simulink model "SingleWksWithTimeBasedFailures"  (R2015a)
settings: Solver=ode45  StartTime=0.0  StopTime=100000  RelTol=1e-3
InitFcn:
  | se_randomizeseeds(gcs, 'Mode', 'All')
undefined symbols (not defined in the file): se_randomizeseeds
libraries: simeventslib x8
settings Model: CovSFcnEnable=off  Creator=gthiers3  LastModifiedBy=gthiers3
settings DebuggingCC: SolverPrmCheckMsg=warning

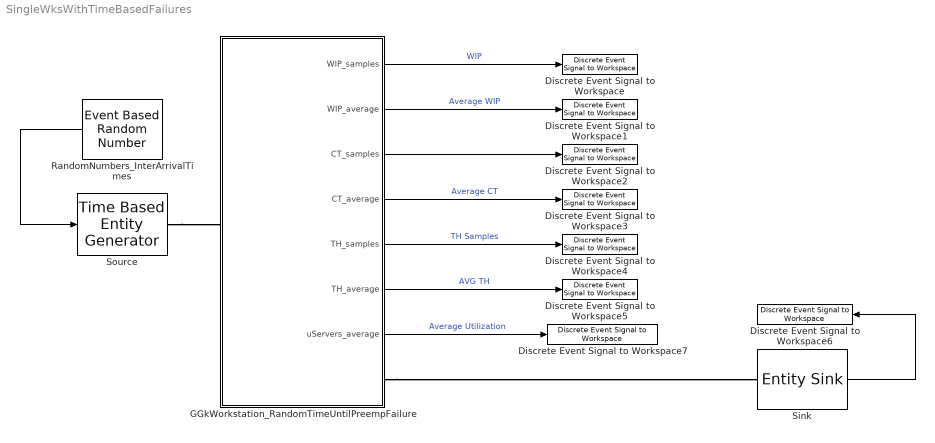
== system SingleWksWithTimeBasedFailures ==
  Discrete Event Signal to Workspace : simeventslib/SimEvents Sinks/Discrete Event Signal to Workspace  VariableName=WIP_samples  SaveFormat=Structure With Time  isMonitorOnly=off  isRecordIC=off
  Discrete Event Signal to Workspace1 : simeventslib/SimEvents Sinks/Discrete Event Signal to Workspace  VariableName=WIP_average  SaveFormat=Structure With Time  isMonitorOnly=off  isRecordIC=off
  Discrete Event Signal to Workspace2 : simeventslib/SimEvents Sinks/Discrete Event Signal to Workspace  VariableName=CT_samples  SaveFormat=Structure With Time  isMonitorOnly=off  isRecordIC=off
  Discrete Event Signal to Workspace3 : simeventslib/SimEvents Sinks/Discrete Event Signal to Workspace  VariableName=CT_average  SaveFormat=Structure With Time  isMonitorOnly=off  isRecordIC=off
  Discrete Event Signal to Workspace4 : simeventslib/SimEvents Sinks/Discrete Event Signal to Workspace  VariableName=TH_samples  SaveFormat=Structure With Time  isMonitorOnly=off  isRecordIC=off
  Discrete Event Signal to Workspace5 : simeventslib/SimEvents Sinks/Discrete Event Signal to Workspace  VariableName=TH_average  SaveFormat=Structure With Time  isMonitorOnly=off  isRecordIC=off
  Discrete Event Signal to Workspace6 : simeventslib/SimEvents Sinks/Discrete Event Signal to Workspace  VariableName=nDepartures  SaveFormat=Structure With Time  isMonitorOnly=off  isRecordIC=off
  Discrete Event Signal to Workspace7 : simeventslib/SimEvents Sinks/Discrete Event Signal to Workspace  VariableName=uServers_average  SaveFormat=Structure With Time  isMonitorOnly=off  isRecordIC=off
  GGkWorkstation_RandomTimeUntilPreempFailure : Subsystem  InitFcn=se_randomizeseeds(gcs, 'Mode', 'All')
      settings: CopyFcn=set_param(gcb, 'LinkStatus', 'none');
  RandomNumbers_InterArrivalTimes : EventBasedRandomNumber  meanExp=25  scaleGam=10  meanNorm=100  stdNorm=eps  Seed=41684
  Sink : EntitySink  StatNumberArrived=on
  Source : TimeBasedEntityGenerator  GenerateEntitiesUpon=Intergeneration time from port t
  wires:
  RandomNumbers_InterArrivalTimes/1 -> Source/1
  GGkWorkstation_RandomTimeUntilPreempFailure/1(WIP_samples) -> Discrete Event Signal to Workspace/1  "WIP"
  GGkWorkstation_RandomTimeUntilPreempFailure/2(WIP_average) -> Discrete Event Signal to Workspace1/1  "Average WIP"
  GGkWorkstation_RandomTimeUntilPreempFailure/3(CT_samples) -> Discrete Event Signal to Workspace2/1
  GGkWorkstation_RandomTimeUntilPreempFailure/4(CT_average) -> Discrete Event Signal to Workspace3/1  "Average CT"
  GGkWorkstation_RandomTimeUntilPreempFailure/7(uServers_average) -> Discrete Event Signal to Workspace7/1  "Average Utilization"
  GGkWorkstation_RandomTimeUntilPreempFailure/6(TH_average) -> Discrete Event Signal to Workspace5/1  "AVG TH"
  GGkWorkstation_RandomTimeUntilPreempFailure/5(TH_samples) -> Discrete Event Signal to Workspace4/1  "TH Samples"
  Sink/1 -> Discrete Event Signal to Workspace6/1
  connections:
  Source/RConn1 -- GGkWorkstation_RandomTimeUntilPreempFailure/LConn1
  GGkWorkstation_RandomTimeUntilPreempFailure/RConn1 -- Sink/LConn1

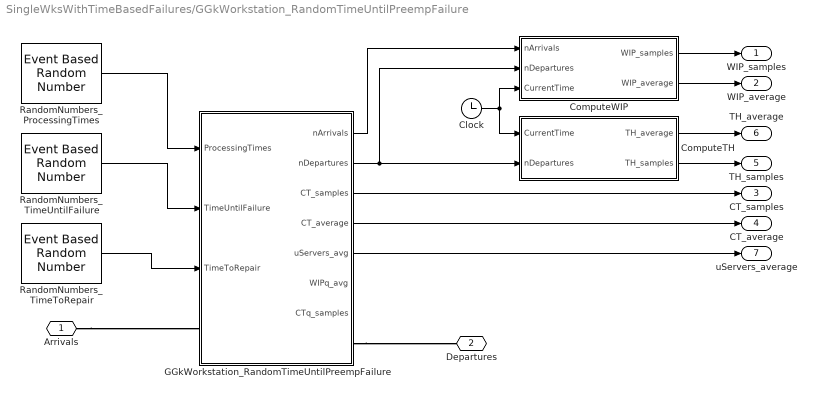
== system SingleWksWithTimeBasedFailures/GGkWorkstation_RandomTimeUntilPreempFailure ==
  Clock : Clock
  ComputeTH : Subsystem
  ComputeWIP : Subsystem
  GGkWorkstation_RandomTimeUntilPreempFailure : Subsystem  mask{NumberOfServers=1}
      mask prompts: NumberOfServers "Number of servers:"
      mask TypeOptions NumberOfServers: N-Server/NumberOfServers
      mask DialogControl DescTextVar Prompt: GG1 Workstation, with random time intervals until preemptive failure and random repair times.  Timing is consistent with Hopp & Spearman’s model, in that the time-until-failure clock stops during repair.
  RandomNumbers_ProcessingTimes : EventBasedRandomNumber  Distribution=Triangular  meanExp=15  minUnif=40  maxUnif=40  pOneBern=40  pSuccessBino=40  numTrialBino=40  minTri=5  maxTri=25  modeTri=15  thresholdGam=40  scaleGam=40  shapeGam=40  meanNorm=95  stdNorm=eps  pSuccessGeo=40  meanPoiss=40  thresholdLogn=40  scaleLogn=40  shapeLogn=40  thresholdLogl=40  scaleLogl=40  minBeta=40  maxBeta=40  shape1Beta=40  shape2Beta=40  minUnid=40  maxUnid=40  numValueUnid=40  thresholdWbl=40  scaleWbl=40  shapeWbl=40  valueVecCont=40  cdfVecCont=40  valueVecDisc=40  probVecDisc=40  Seed=32033
  RandomNumbers_TimeToRepair : EventBasedRandomNumber  Distribution=Gaussian (normal)  meanExp=248  minUnif=40  maxUnif=40  pOneBern=40  pSuccessBino=40  numTrialBino=40  minTri=40  maxTri=40  modeTri=40  scaleGam=20  meanNorm=40  stdNorm=eps  pSuccessGeo=40  meanPoiss=40  thresholdLogn=40  scaleLogn=40  shapeLogn=40  thresholdLogl=40  scaleLogl=40  minBeta=40  maxBeta=40  shape1Beta=40  shape2Beta=40  minUnid=40  maxUnid=40  numValueUnid=40  thresholdWbl=40  scaleWbl=40  shapeWbl=40  valueVecCont=40  cdfVecCont=40  probVecDisc=[0 1]  Seed=35250
  RandomNumbers_TimeUntilFailure : EventBasedRandomNumber  meanExp=120  minUnif=40  maxUnif=40  pOneBern=40  pSuccessBino=40  numTrialBino=40  minTri=744  maxTri=744  modeTri=744  scaleGam=166.6667  shapeGam=0.72  meanNorm=1000  stdNorm=1.4901e-08  pSuccessGeo=40  meanPoiss=40  thresholdLogn=40  scaleLogn=40  shapeLogn=40  thresholdLogl=40  scaleLogl=40  minBeta=40  maxBeta=40  shape1Beta=40  shape2Beta=40  minUnid=40  maxUnid=40  numValueUnid=40  thresholdWbl=40  scaleWbl=40  shapeWbl=40  valueVecCont=40  cdfVecCont=40  valueVecDisc=40  probVecDisc=40  Seed=38467
  Arrivals : PMIOPort  Port=1  Side=Left
  Departures : PMIOPort  Port=2  Side=Right
  WIP_samples : Outport
  WIP_average : Outport  Port=2
  CT_samples : Outport  Port=3
  CT_average : Outport  Port=4
  TH_samples : Outport  Port=5
  TH_average : Outport  Port=6
  uServers_average : Outport  Port=7
  wires:
  RandomNumbers_ProcessingTimes/1 -> GGkWorkstation_RandomTimeUntilPreempFailure/1(ProcessingTimes)
  GGkWorkstation_RandomTimeUntilPreempFailure/5(uServers_avg) -> uServers_average/1
  GGkWorkstation_RandomTimeUntilPreempFailure/2(nDepartures) -> ComputeTH/2(nDepartures), ComputeWIP/2(nDepartures)
  GGkWorkstation_RandomTimeUntilPreempFailure/3(CT_samples) -> CT_samples/1
  GGkWorkstation_RandomTimeUntilPreempFailure/4(CT_average) -> CT_average/1
  ComputeWIP/1(WIP_samples) -> WIP_samples/1
  ComputeWIP/2(WIP_average) -> WIP_average/1
  GGkWorkstation_RandomTimeUntilPreempFailure/1(nArrivals) -> ComputeWIP/1(nArrivals)
  Clock/1 -> ComputeWIP/3(CurrentTime), ComputeTH/1(CurrentTime)
  ComputeTH/1(TH_average) -> TH_average/1
  ComputeTH/2(TH_samples) -> TH_samples/1
  RandomNumbers_TimeUntilFailure/1 -> GGkWorkstation_RandomTimeUntilPreempFailure/2(TimeUntilFailure)
  RandomNumbers_TimeToRepair/1 -> GGkWorkstation_RandomTimeUntilPreempFailure/3(TimeToRepair)
  connections:
  GGkWorkstation_RandomTimeUntilPreempFailure/RConn1 -- Departures/RConn1
  Arrivals/RConn1 -- GGkWorkstation_RandomTimeUntilPreempFailure/LConn1

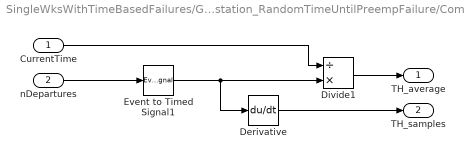
== system SingleWksWithTimeBasedFailures/GGkWorkstation_RandomTimeUntilPreempFailure/ComputeTH ==
  CurrentTime : Inport
  nDepartures : Inport  Port=2
  Derivative : Derivative
  Divide1 : Product  Inputs=/*
  Event to Timed Signal1 : EventToTimedSignal
  TH_average : Outport
  TH_samples : Outport  Port=2
  wires:
  CurrentTime/1 -> Divide1/1
  Event to Timed Signal1/1 -> Derivative/1, Divide1/2
  Divide1/1 -> TH_average/1
  Derivative/1 -> TH_samples/1
  nDepartures/1 -> Event to Timed Signal1/1

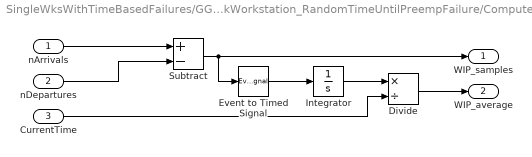
== system SingleWksWithTimeBasedFailures/GGkWorkstation_RandomTimeUntilPreempFailure/ComputeWIP ==
  nArrivals : Inport
  nDepartures : Inport  Port=2
  CurrentTime : Inport  Port=3
  Divide : Product  Inputs=*/
  Event to Timed Signal : EventToTimedSignal
  Integrator : Integrator
  Subtract : Sum  Inputs=+-
  WIP_samples : Outport
  WIP_average : Outport  Port=2
  wires:
  Subtract/1 -> WIP_samples/1, Event to Timed Signal/1
  Event to Timed Signal/1 -> Integrator/1
  Divide/1 -> WIP_average/1
  Integrator/1 -> Divide/1
  nArrivals/1 -> Subtract/1
  nDepartures/1 -> Subtract/2
  CurrentTime/1 -> Divide/2

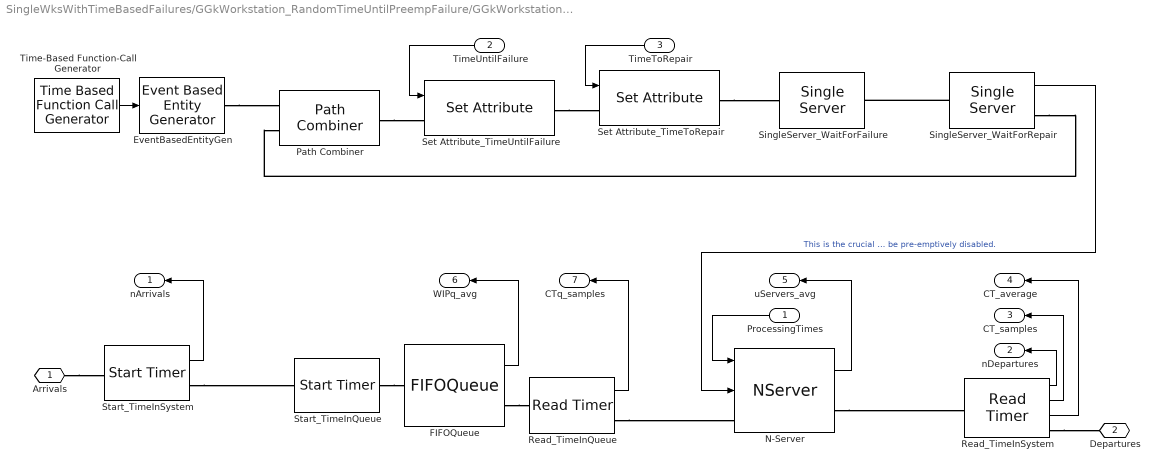
== system SingleWksWithTimeBasedFailures/GGkWorkstation_RandomTimeUntilPreempFailure/GGkWorkstation_RandomTimeUntilPreempFailure ==
  ProcessingTimes : Inport
  TimeUntilFailure : Inport  Port=2
  TimeToRepair : Inport  Port=3
  EventBasedEntityGen : EventBasedEntityGenerator  GenerateEntitiesUpon=Function call from port fcn
  FIFOQueue : FIFOQueue  Capacity=Inf  StatAverageQueueLength=on
      settings: OutputPortMap=o3
  N-Server : NServer  NumberOfServers=NumberOfServers  ServiceTimeFrom=Signal port t  AllowServiceControl=on  BlockWhileSignalOn=on  StatUtilization=on
      settings: InputPortMap=u0,u1  OutputPortMap=o5
  Path Combiner : PathCombiner  NumberInputPorts=2
  Read_TimeInQueue : ReadTimer  TimerTag=TimeInQueue  StatTimeElapsed=on
      settings: OutputPortMap=o2
  Read_TimeInSystem : ReadTimer  TimerTag=TimeInSystem  StatNumberDeparted=on  StatTimeElapsed=on  StatAverageTimeElapsed=on
      settings: OutputPortMap=o0,o2,o3
  Set Attribute_TimeToRepair : SetAttribute  AttributeName=TimeToRepair  AttributeFrom=Signal port  EvaluatedAttributeValue={ []}
  Set Attribute_TimeUntilFailure : SetAttribute  AttributeName=TimeUntilFailure  AttributeFrom=Signal port  EvaluatedAttributeValue={ []}
  SingleServer_WaitForFailure : SingleServer  ServiceTimeFrom=Attribute  AttributeName=TimeUntilFailure
  SingleServer_WaitForRepair : SingleServer  ServiceTimeFrom=Attribute  AttributeName=TimeToRepair  StatNumberInBlock=on
      settings: OutputPortMap=o1
  Start_TimeInQueue : StartTimer  TimerTag=TimeInQueue  TimerStartedOption=Restart
  Start_TimeInSystem : StartTimer  TimerTag=TimeInSystem  TimerStartedOption=Restart  StatNumberDeparted=on
  Time-Based Function-Call Generator : TimeBasedFunctionCallGenerator  EventGenerationMode=Only at simulation start
  Arrivals : PMIOPort  Port=1  Side=Left
  Departures : PMIOPort  Port=2  Side=Right
  nArrivals : Outport
  nDepartures : Outport  Port=2
  CT_samples : Outport  Port=3
  CT_average : Outport  Port=4
  uServers_avg : Outport  Port=5
  WIPq_avg : Outport  Port=6
  CTq_samples : Outport  Port=7
  wires:
  Read_TimeInSystem/2 -> CT_samples/1
  N-Server/1 -> uServers_avg/1
  Read_TimeInQueue/1 -> CTq_samples/1
  FIFOQueue/1 -> WIPq_avg/1
  Start_TimeInSystem/1 -> nArrivals/1
  Read_TimeInSystem/1 -> nDepartures/1
  ProcessingTimes/1 -> N-Server/1
  Read_TimeInSystem/3 -> CT_average/1
  TimeToRepair/1 -> Set Attribute_TimeToRepair/1
  Time-Based Function-Call Generator/1 -> EventBasedEntityGen/1
  TimeUntilFailure/1 -> Set Attribute_TimeUntilFailure/1
  SingleServer_WaitForRepair/1 -> N-Server/2  "This is the crucial blocking signal. When > 0, the N-Server will be pre-emptively disabled."
  connections:
  Arrivals/RConn1 -- Start_TimeInSystem/LConn1
  N-Server/RConn1 -- Read_TimeInSystem/LConn1
  FIFOQueue/RConn1 -- Read_TimeInQueue/LConn1
  Start_TimeInSystem/RConn1 -- Start_TimeInQueue/LConn1
  Read_TimeInSystem/RConn1 -- Departures/RConn1
  Read_TimeInQueue/RConn1 -- N-Server/LConn1
  Start_TimeInQueue/RConn1 -- FIFOQueue/LConn1
  Path Combiner/RConn1 -- Set Attribute_TimeUntilFailure/LConn1
  SingleServer_WaitForRepair/LConn1 -- SingleServer_WaitForFailure/RConn1
  EventBasedEntityGen/RConn1 -- Path Combiner/LConn1
  SingleServer_WaitForRepair/RConn1 -- Path Combiner/LConn2
  Set Attribute_TimeUntilFailure/RConn1 -- Set Attribute_TimeToRepair/LConn1
  Set Attribute_TimeToRepair/RConn1 -- SingleServer_WaitForFailure/LConn1
